simulink model "Problem2"  (R2020a)
settings: Solver=VariableStepAuto  StartTime=0.0  StopTime=10.0  RelTol=1e-3
settings Model: Creator=tanu  LastModifiedBy=tanu

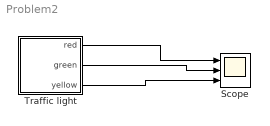
== system Problem2 ==
  Scope : Scope  NumInputPorts=3
  Traffic light : Stateflow chart  TreatAsAtomicUnit=on
      settings: PortSchema="{\"entries\":[{\"content\":{\"sides\":[{\"content\":{\"connectorIds\":[]},\"type\":\"ConnectorPlacement.EquallySpacedRectSide\",\"uuid\":\"7908a64d-f54a-47f3-9c30-64c16fd9ea89\"},{\"content\":{\"connectorIds\":[\"Out2\",\"Out1\",\"Out3\"],\"side\":\"RIGHT\"},\"type\":\"ConnectorPlacement.EquallySpacedRectSide\",\"uuid\":\"22914987-d09b-464a-ac4a-1c04fe56a1f1\"},{\"content\":{\"connectorIds\":[],\"side\":\"TOP\"},\"type\":\"ConnectorPlacement.EquallySpacedRectSide\",\"uuid\":\"57176934-5f65-47bd-8005-0c5537b5a047\"}]},\"type\":\"ConnectorPlacement.EquallySpacedConnector\",\"uuid\":\"9fe24e74-e534-40c9-91b0-f46a3029d52a\"}],\"packageUris\":[\"http://schema.mathworks.com/mf0/Connector/19700101\"],\"version\":\"1.0\"}"
  wires:
  Traffic light/2(red) -> Scope/1
  Traffic light/1(green) -> Scope/2
  Traffic light/3(yellow) -> Scope/3

== stateflow chart Problem2/Traffic light ==
  state Stop
    entry:
    red = 1;
    yellow = 0;
    green = 0;
  state PrepareToStop
    entry:
    red = 0;
    yellow = 1;
    green = 0;
  state Go
    entry:
    red = 0;
    yellow = 0;
    green = 1;
  (default) -> Stop
  Stop -> (junction 11)
  (junction 11) -> (junction 4) : after(3,sec)
  PrepareToStop -> Stop : after(3,sec)
  Go -> PrepareToStop : after(10,sec)
  (junction 4) -> Go
  data: green output; red output; yellow output
